simulink model "SB11_enabled_done"  (R2024b)
settings: Solver=FixedStepDiscrete  StartTime=0.0  StopTime=20  FixedStep=0.05  RelTol=1e-3
settings Model: Creator=admin  LastModifiedBy=admin

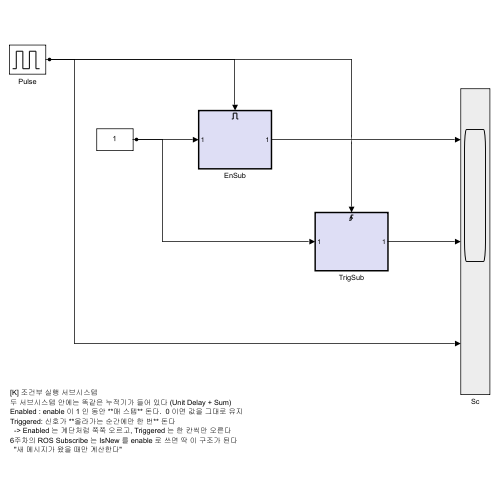
[thumbnail: Simulink's stored preview of the top-level diagram]
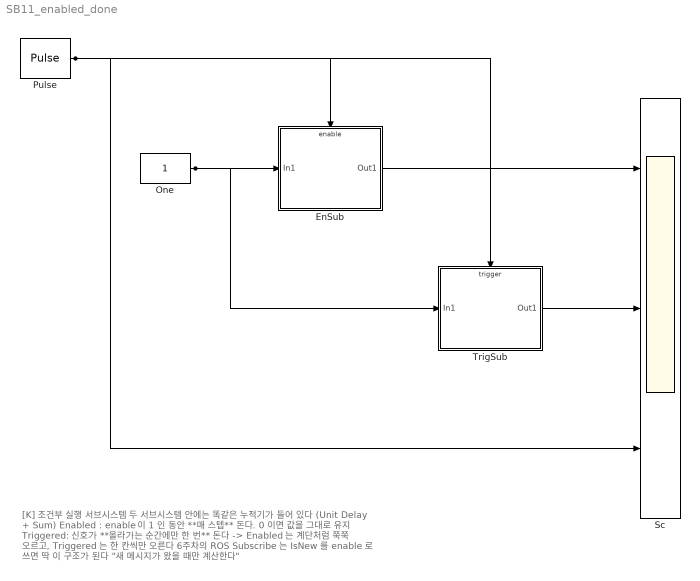
== system SB11_enabled_done ==
  note: [K] 조건부 실행 서브시스템
      | 두 서브시스템 안에는 똑같은 누적기가 들어 있다 (Unit Delay + Sum)
      | Enabled : enable 이 1 인 동안 **매 스텝** 돈다.  0 이면 값을 그대로 유지
      | Triggered: 신호가 **올라가는 순간에만 한 번** 돈다
      |   -> Enabled 는 계단처럼 쭉쭉 오르고, Triggered 는 한 칸씩만 오른다
      | 6주차의 ROS Subscribe 는 IsNew 를 enable 로 쓰면 딱 이 구조가 된다
      |   "새 메시지가 왔을 때만 계산한다"
  EnSub : Subsystem  TreatAsAtomicUnit=on
  One : Constant
  Pulse : DiscretePulseGenerator  PulseType=Time based  Period=4  PulseWidth=50  SampleTime=0.05
  Sc : Scope  NumInputPorts=3
  TrigSub : Subsystem  TreatAsAtomicUnit=on
  wires:
  One/1 -> EnSub/1(In1), TrigSub/1(In1)
  Pulse/1 -> EnSub/Enable, TrigSub/Trigger, Sc/3
  EnSub/1(Out1) -> Sc/1
  TrigSub/1(Out1) -> Sc/2

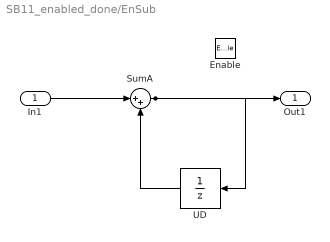
== system SB11_enabled_done/EnSub ==
  In1 : Inport
  Enable : EnablePort
  SumA : Sum  Inputs=|++
  UD : UnitDelay  SampleTime=-1  HasFrameUpgradeWarning=on
  Out1 : Outport
  wires:
  In1/1 -> SumA/1
  SumA/1 -> Out1/1, UD/1
  UD/1 -> SumA/2

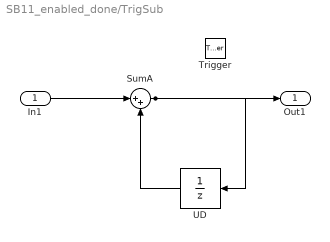
== system SB11_enabled_done/TrigSub ==
  In1 : Inport
  Trigger : TriggerPort  VariantControl=(inherit)
  SumA : Sum  Inputs=|++
  UD : UnitDelay  SampleTime=-1  HasFrameUpgradeWarning=on
  Out1 : Outport
  wires:
  In1/1 -> SumA/1
  SumA/1 -> Out1/1, UD/1
  UD/1 -> SumA/2
